simulink model "Tarea4_LuminosidadHAcumulativo"  (R2022b)
settings: Solver=VariableStepAuto  StartTime=0.0  StopTime=10.0  RelTol=1e-3
undefined symbols (not defined in the file): concatena1, none, Rec, SDTV, videoinput
libraries: visionconversions x2, visionstatistics x1, visiontextngfix x1, imaqlib x1, visionsources x1
settings Model: Creator=esteb  LastModifiedBy=esteb

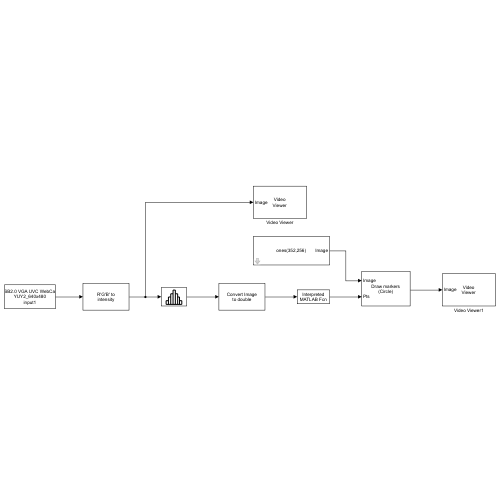
[thumbnail: Simulink's stored preview of the top-level diagram]
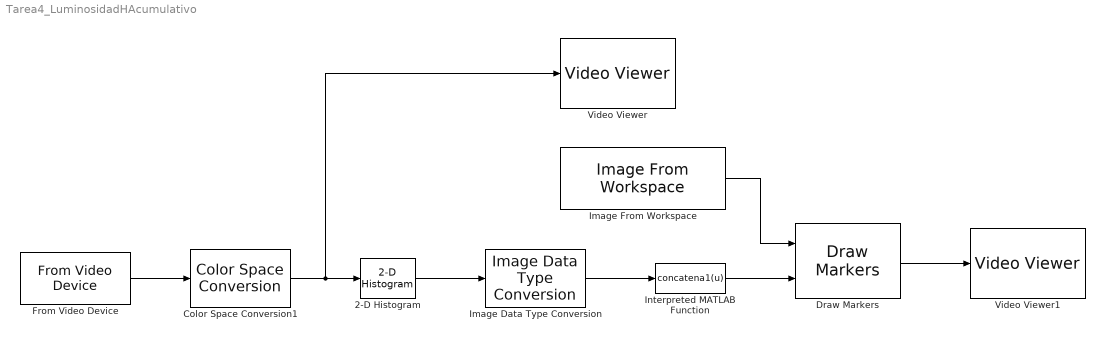
== system Tarea4_LuminosidadHAcumulativo ==
  2-D Histogram : visionstatistics/2-D Histogram  umin=0  umax=1  nbins=256  operateOver=Entire input  normalized=on  run=off  reset=on  trigtype=None  Dimension=1  colComp=on  roundingMode=Floor  overflowMode=off
  Color Space Conversion1 : visionconversions/Color Space  Conversion  conversion=Obsolete  conversionActive=R'G'B' to intensity  wp_str=D65  rec=Rec. 601 (SDTV)  sys=1125/60/2:1  imagePorts=One multidimensional signal
  Draw Markers : visiontextngfix/Draw Markers  shape=Circle  size=3  fill=off  fillClrSource=Specify via dialog  display=Black  intensity=200  color=[200 255 100]  opacity=0.6  viewport=Entire image  antialiasing=off  inType=Obsolete  imagePorts=One multidimensional signal  roundingMode=Floor  overflowMode=off  memoryMode=Specify word length  memoryWordLength=16  memoryFracLength=15  prodOutputMode=Binary point scaling  prodOutputWordLength=32  prodOutputFracLength=14
  From Video Device : imaqlib/From Video Device  DeviceMenu=winvideo 1 (USB2.0 VGA UVC WebCam)  Device=winvideo 1 (USB2.0 VGA UVC WebCam)  ObjConstructor=videoinput('winvideo', 1)  VideoFormatMenu=YUY2_640x480  VideoFormat=YUY2_640x480  VideoSource=input1  ROIPosition=[0 0 480 640]  EnableHWTrigger=off  TriggerConfiguration=none/none  SampleTime=1/30  OutputPortsMode=One multidimensional signal  DataType=single  CanDoHWTrigger=no  ReturnedColorSpace=YCbCr  BlockHandle=4.0002  ROIWidth=640  ROIHeight=480  ROIColumn=0  ROIRow=0  EngXMLPath=C:\Program Files\MATLAB\R2022b\toolbox\imaq\imaq\private  DevXMLPath=C:\ProgramData\MATLAB\SupportPackages\R2022b\toolbox\imaq\supportpackages\genericvideo\adaptor\win64  EngLibPath=C:\Program Files\MATLAB\R2022b\toolbox\imaq\imaqblks\imaqmex\win64  ColorSpace=YCbCr  BayerSensorAlignment=grbg  ImaqMode=off
  Image Data Type Conversion : visionconversions/Image Data Type Conversion  outDT=double  isSigned=on  wordLen=16  numFracBits=0
  Image From Workspace : visionsources/Image From Workspace  Tag=vipblks_nd  ImageValue=ones(352,256)  Ts=inf  imagePorts=One multidimensional signal  OutPortLabels=R|G|B  ImageDataType=Inherit from 'Value'  Signed=on  WordLength=16  sdImageDataType=sfix(16)  FractionLengthMode=User-defined  FractionLength=15
  Interpreted MATLAB Function : MATLABFcn  MATLABFcn=concatena1(u)  Output1D=off
  Video Viewer : VideoViewer  FigPos=[559 583 418 304]
  Video Viewer1 : VideoViewer  FigPos=[559 583 418 304]
  wires:
  Image Data Type Conversion/1 -> Interpreted MATLAB Function/1
  Image From Workspace/1 -> Draw Markers/1
  Draw Markers/1 -> Video Viewer1/1
  Interpreted MATLAB Function/1 -> Draw Markers/2
  From Video Device/1 -> Color Space Conversion1/1
  Color Space Conversion1/1 -> Video Viewer/1, 2-D Histogram/1
  2-D Histogram/1 -> Image Data Type Conversion/1
